simulink model "Simulator2019a"  (R2019a)
settings: Solver=FixedStepAuto  StartTime=0.0  StopTime=20  FixedStep=dt  RelTol=1e-3
model workspace (MAT data in the model file):
  s000 = 0
values from neighbouring files (symbols this model uses):
  Ixx = aircraft_data(53)    [main_code.m]    (also in untitled4.m; untitled5.m)
  Iyy = aircraft_data(54)    [main_code.m]    (also in untitled4.m; untitled5.m)
  Izz = aircraft_data(55)    [main_code.m]    (also in untitled4.m; untitled5.m)
  M_0 = [0; 0; 0]    [main_code.m]    (also in untitled4.m; untitled5.m)
  Matrix_states = [Xu, 0, Xw, 0, 0, 0, 0 ... (first row only)    [main_code.m]    (also in untitled4.m)
  w_dot0 = Vb_dot_0(3)    [untitled5.m]
undefined symbols (not defined in the file or in its folder): Fg_0, g, K, m, Matrix_Controllers, s0
libraries: dspsigops x3, simulink_extras x1, SignalEditorBlockLib x1, shared6dof x1, aerolibasang x1
settings Model: Creator=Administrator  LastModifiedBy=Ahmed Essam

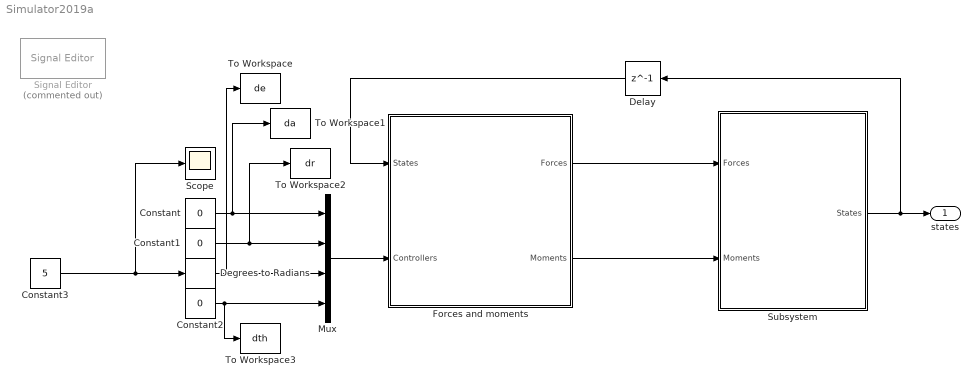
== system Simulator2019a ==
  Constant : Constant  Value=0
  Constant1 : Constant  Value=0
  Constant2 : Constant  Value=0
  Constant3 : Constant  Value=5
  Degrees to Radians : simulink_extras/Transformations/Degrees to Radians
  Delay : Delay  DelayLength=1  InitialCondition=K
  Forces and moments : Subsystem
  Mux : Mux
  Scope : Scope
  Signal Editor : SignalEditorBlockLib/Signal Editor  Commented=on  FileName=Elevator.mat  ActiveScenario=Scenario  ActiveSignal=dE  IsBus=off  OutputBusObjectStr=Bus: BusObject  SampleTime=0  Interpolate=off  ZeroCross=off  OutputAfterFinalValue=Setting to zero  Unit=inherit  PreserveSignalName=on
  Subsystem : Subsystem
  To Workspace : ToWorkspace  VariableName=de  SampleTime=-1
      settings: Save2DSignal=2-D array (concatenate along first dimension)
  To Workspace1 : ToWorkspace  VariableName=da  SampleTime=-1
      settings: Save2DSignal=2-D array (concatenate along first dimension)
  To Workspace2 : ToWorkspace  VariableName=dr  SampleTime=-1
      settings: Save2DSignal=2-D array (concatenate along first dimension)
  To Workspace3 : ToWorkspace  VariableName=dth  SampleTime=-1
      settings: Save2DSignal=2-D array (concatenate along first dimension)
  states : Outport  VectorParamsAs1DForOutWhenUnconnected=on
  wires:
  Subsystem/1(States) -> Delay/1, states/1
  Forces and moments/1(Forces) -> Subsystem/1(Forces)
  Forces and moments/2(Moments) -> Subsystem/2(Moments)
  Mux/1 -> Forces and moments/2(Controllers)
  Delay/1 -> Forces and moments/1(States)
  Constant/1 -> To Workspace1/1, Mux/1
  Constant1/1 -> To Workspace2/1, Mux/2
  Constant2/1 -> To Workspace3/1, Mux/4
  Degrees to Radians/1 -> To Workspace/1, Mux/3
  Constant3/1 -> Scope/1, Degrees to Radians/1

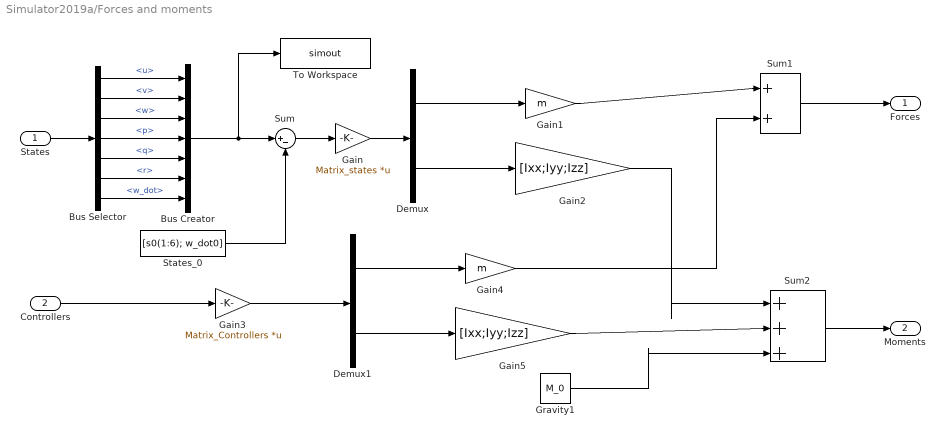
== system Simulator2019a/Forces and moments ==
  States : Inport
  Controllers : Inport  Port=2
  Bus Creator : BusCreator  Inputs=7
  Bus Selector : BusSelector  OutputSignals=u,v,w,p,q,r,w_dot
  Demux : Demux  Outputs=2
  Demux1 : Demux  Outputs=2
  Gain : Gain  Gain=Matrix_states  Multiplication=Matrix(K*u)
  Gain1 : Gain  Gain=m
  Gain2 : Gain  Gain=[Ixx;Iyy;Izz]
  Gain3 : Gain  Gain=Matrix_Controllers  Multiplication=Matrix(K*u)
  Gain4 : Gain  Gain=m
  Gain5 : Gain  Gain=[Ixx;Iyy;Izz]
  Gravity1 : Constant  Value=M_0
  States_0 : Constant  Value=[s0(1:6); w_dot0]
  Sum : Sum  Inputs=|+-
  Sum1 : Sum  Inputs=|++
  Sum2 : Sum  Inputs=|+++
  To Workspace : ToWorkspace  VariableName=simout  SampleTime=-1
  Forces : Outport  VectorParamsAs1DForOutWhenUnconnected=on
  Moments : Outport  Port=2  VectorParamsAs1DForOutWhenUnconnected=on
  wires:
  Gain1/1 -> Sum1/1
  Bus Selector/6 -> Bus Creator/6  "<r>"
  Demux/2 -> Gain2/1
  Gain/1 -> Demux/1
  Gain3/1 -> Demux1/1
  Bus Selector/4 -> Bus Creator/4  "<p>"
  Sum2/1 -> Moments/1
  Sum/1 -> Gain/1
  Bus Selector/2 -> Bus Creator/2  "<v>"
  States_0/1 -> Sum/2
  Gain4/1 -> Sum1/2
  Bus Creator/1 -> To Workspace/1, Sum/1
  Bus Selector/1 -> Bus Creator/1  "<u>"
  Bus Selector/5 -> Bus Creator/5  "<q>"
  Controllers/1 -> Gain3/1
  Gravity1/1 -> Sum2/3
  Bus Selector/3 -> Bus Creator/3  "<w>"
  Bus Selector/7 -> Bus Creator/7  "<w_dot>"
  Demux/1 -> Gain1/1
  Demux1/1 -> Gain4/1
  Demux1/2 -> Gain5/1
  States/1 -> Bus Selector/1
  Gain2/1 -> Sum2/1
  Gain5/1 -> Sum2/2
  Sum1/1 -> Forces/1

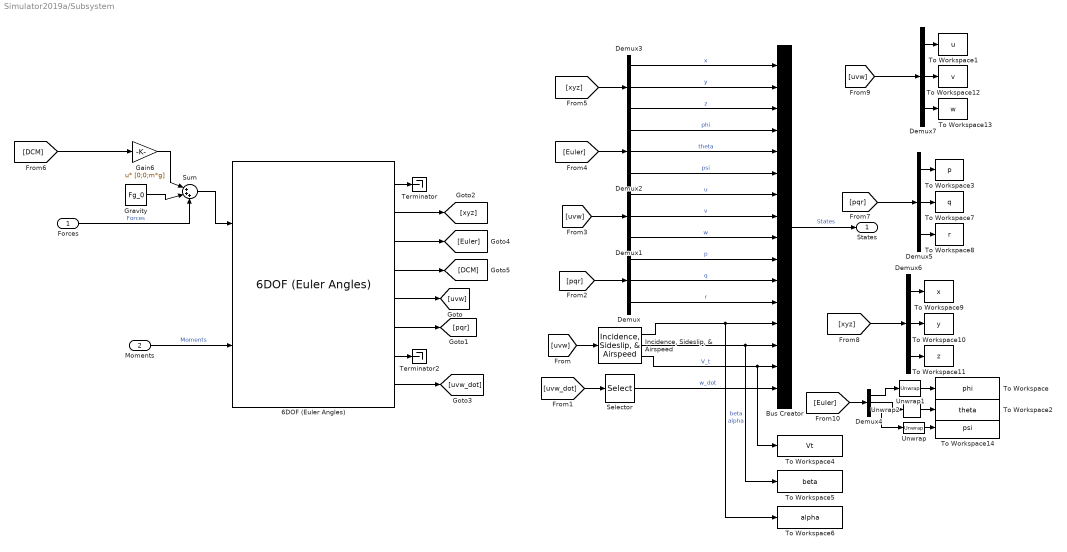
== system Simulator2019a/Subsystem ==
  Forces : Inport
  Moments : Inport  Port=2
  6DOF (Euler Angles) : shared6dof/6DOF (Euler Angles)  units=English (Velocity in ft/s)  mtype=Fixed  rep=Euler Angles  xme_0=s0(10:12)  Vm_0=s0(1:3)  eul_0=s0(7:9)  pm_0=s0(4:6)  mass_0=m  mass_e=0.5  mass_f=2.0  inertia=I  inertia_e=eye(3)  inertia_f=2*eye(3)  k_quat=1.0  vre_flag=on  abi_flag=off  aMode=0  xme_statename=''  Vm_statename=''  eul_statename=''  quat_statename=''  pm_statename=''  mass_statename=''
      settings: SourceProductBaseCode=AE,PW,DR,MT,UV,VE
  Bus Creator : BusCreator  Inputs=16
  Demux{,1..7} (8 alike) : Demux  Outputs=3
  Gain6 : Gain  Gain=[0;0;m*g]  Multiplication=Matrix(u*K)
  Gravity : Constant  Value=Fg_0
  "Incidence, Sideslip, & Airspeed" : aerolibasang/Incidence, Sideslip, & Airspeed
  Selector : Selector  InputPortWidth=3  IndexOptions=Index vector (dialog)  Indices=3  OutputSizes=1
  Sum : Sum  Inputs=|+++
  Terminator : Terminator
  Terminator2 : Terminator
  To Workspace : ToWorkspace  VariableName=phi  SampleTime=-1
      settings: Save2DSignal=2-D array (concatenate along first dimension)
  To Workspace1 : ToWorkspace  VariableName=u  SampleTime=-1
      settings: Save2DSignal=2-D array (concatenate along first dimension)
  To Workspace10 : ToWorkspace  VariableName=y  SampleTime=-1
      settings: Save2DSignal=2-D array (concatenate along first dimension)
  To Workspace11 : ToWorkspace  VariableName=z  SampleTime=-1
      settings: Save2DSignal=2-D array (concatenate along first dimension)
  To Workspace12 : ToWorkspace  VariableName=v  SampleTime=-1
      settings: Save2DSignal=2-D array (concatenate along first dimension)
  To Workspace13 : ToWorkspace  VariableName=w  SampleTime=-1
      settings: Save2DSignal=2-D array (concatenate along first dimension)
  To Workspace14 : ToWorkspace  VariableName=psi  SampleTime=-1
      settings: Save2DSignal=2-D array (concatenate along first dimension)
  To Workspace2 : ToWorkspace  VariableName=theta  SampleTime=-1
      settings: Save2DSignal=2-D array (concatenate along first dimension)
  To Workspace3 : ToWorkspace  VariableName=p  SampleTime=-1
      settings: Save2DSignal=2-D array (concatenate along first dimension)
  To Workspace4 : ToWorkspace  VariableName=Vt  SampleTime=-1
  To Workspace5 : ToWorkspace  VariableName=beta  SampleTime=-1
  To Workspace6 : ToWorkspace  VariableName=alpha  SampleTime=-1
  To Workspace7 : ToWorkspace  VariableName=q  SampleTime=-1
      settings: Save2DSignal=2-D array (concatenate along first dimension)
  To Workspace8 : ToWorkspace  VariableName=r  SampleTime=-1
      settings: Save2DSignal=2-D array (concatenate along first dimension)
  To Workspace9 : ToWorkspace  VariableName=x  SampleTime=-1
      settings: Save2DSignal=2-D array (concatenate along first dimension)
  Unwrap : dspsigops/Unwrap  tol=pi  InputProcessing=Columns as channels (frame based)  running=off
  Unwrap1 : dspsigops/Unwrap  tol=pi  InputProcessing=Columns as channels (frame based)  running=off
  Unwrap2 : dspsigops/Unwrap  tol=pi  InputProcessing=Columns as channels (frame based)  running=off
  States : Outport  VectorParamsAs1DForOutWhenUnconnected=on
  wires:
  6DOF (Euler Angles)/3 -> [Euler]
  "Incidence, Sideslip, & Airspeed"/1 -> Bus Creator/13, To Workspace6/1  "alpha"
  [xyz] -> Demux3/1
  [uvw_dot] -> Selector/1
  6DOF (Euler Angles)/8 -> [uvw_dot]
  "Incidence, Sideslip, & Airspeed"/2 -> To Workspace5/1, Bus Creator/14  "beta"
  "Incidence, Sideslip, & Airspeed"/3 -> Bus Creator/15, To Workspace4/1  "V_t"
  [uvw] -> Demux1/1
  6DOF (Euler Angles)/1 -> Terminator/1
  [Euler] -> Demux2/1
  Demux/2 -> Bus Creator/11  "q"
  Bus Creator/1 -> States/1  "States"
  6DOF (Euler Angles)/7 -> Terminator2/1
  Demux1/3 -> Bus Creator/9  "w"
  Demux3/1 -> Bus Creator/1  "x"
  Demux/3 -> Bus Creator/12  "r"
  [uvw] -> "Incidence, Sideslip, & Airspeed"/1
  Demux3/3 -> Bus Creator/3  "z"
  Demux3/2 -> Bus Creator/2  "y"
  Forces/1 -> Sum/3  "Forces"
  6DOF (Euler Angles)/4 -> [DCM]
  6DOF (Euler Angles)/2 -> [xyz]
  [pqr] -> Demux/1
  Demux/1 -> Bus Creator/10  "p"
  Selector/1 -> Bus Creator/16  "w_dot"
  Demux1/2 -> Bus Creator/8  "v"
  6DOF (Euler Angles)/6 -> [pqr]
  6DOF (Euler Angles)/5 -> [uvw]
  Moments/1 -> 6DOF (Euler Angles)/2  "Moments"
  Demux1/1 -> Bus Creator/7  "u"
  Demux2/1 -> Bus Creator/4  "phi"
  Demux2/2 -> Bus Creator/5  "theta"
  Demux2/3 -> Bus Creator/6  "psi"
  Gain6/1 -> Sum/1
  Gravity/1 -> Sum/2
  [DCM] -> Gain6/1
  Sum/1 -> 6DOF (Euler Angles)/1
  [pqr] -> Demux5/1
  [Euler] -> Demux4/1
  Demux4/3 -> Unwrap/1
  Demux4/1 -> Unwrap1/1
  Demux4/2 -> Unwrap2/1
  Demux5/1 -> To Workspace3/1
  Demux5/2 -> To Workspace7/1
  Demux5/3 -> To Workspace8/1
  Demux6/2 -> To Workspace10/1
  [xyz] -> Demux6/1
  Demux6/3 -> To Workspace11/1
  Demux6/1 -> To Workspace9/1
  Demux7/2 -> To Workspace12/1
  [uvw] -> Demux7/1
  Demux7/3 -> To Workspace13/1
  Demux7/1 -> To Workspace1/1
  Unwrap2/1 -> To Workspace2/1
  Unwrap/1 -> To Workspace14/1
  Unwrap1/1 -> To Workspace/1
